simulink model "Statefunction"  (R2016a)
settings: Solver=VariableStepAuto  StartTime=0.0  StopTime=100  RelTol=1e-3
libraries: simulink x1
settings Model: Creator=24535  LastModifiedBy=24535

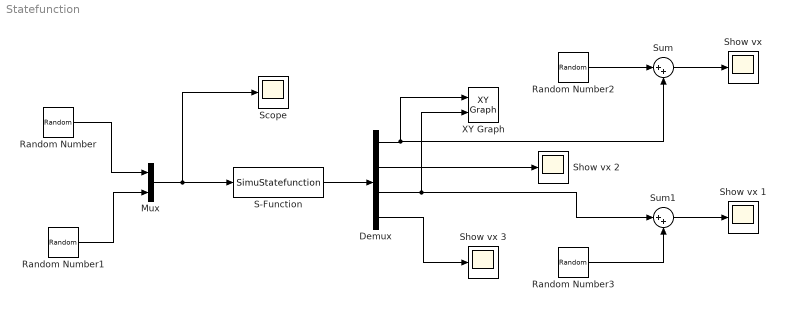
== system Statefunction ==
   Show vx {,1..3} (4 alike) : Scope
  Demux : Demux
  Mux : Mux  Inputs=2
  Random Number : RandomNumber  Variance=0.01  SampleTime=1
  Random Number1 : RandomNumber  Variance=0.09  Seed=3  SampleTime=1
  Random Number2 : RandomNumber  Variance=0.04  SampleTime=1
  Random Number3 : RandomNumber  Variance=0.04  Seed=3  SampleTime=1
  S-Function : S-Function  FunctionName=SimuStatefunction  SFunctionDeploymentMode=off  EnableBusSupport=off
  Scope : Scope
  Sum : Sum  Inputs=|++
  Sum1 : Sum  Inputs=|++
  XY Graph : simulink/Sinks/XY Graph  xmin=0  xmax=600  ymin=0  ymax=600  st=-1
  wires:
  Random Number/1 -> Mux/1
  Random Number1/1 -> Mux/2
  Mux/1 -> Scope/1, S-Function/1
  S-Function/1 -> Demux/1
  Demux/3 -> Sum1/1, XY Graph/2
  Demux/1 -> Sum/2, XY Graph/1
  Sum/1 -> " Show vx "/1
  Random Number2/1 -> Sum/1
  Random Number3/1 -> Sum1/2
  Sum1/1 -> " Show vx 1"/1
  Demux/2 -> " Show vx 2"/1
  Demux/4 -> " Show vx 3"/1
